simulink model "exp4simu"  (R2022b)
settings: Solver=VariableStepAuto  StartTime=0.0  StopTime=10.0  RelTol=1e-3
settings Model: Creator=16033  LastModifiedBy=16033

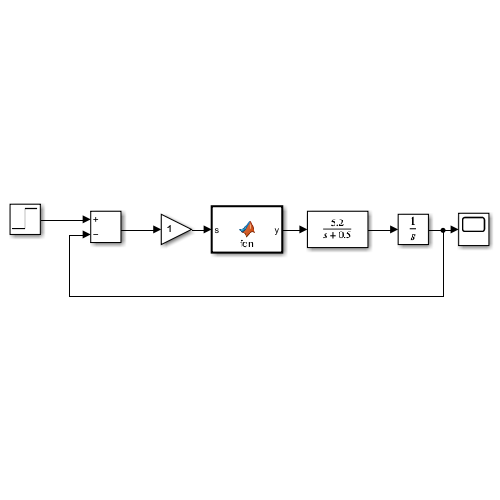
[thumbnail: Simulink's stored preview of the top-level diagram]
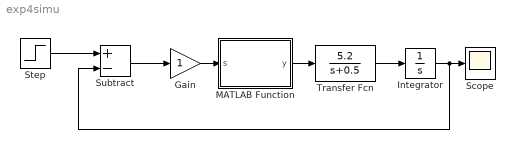
== system exp4simu ==
  Gain : Gain
  Integrator : Integrator
  MATLAB Function : MATLAB Function  TreatAsAtomicUnit=on
  Scope : Scope
  Step : Step  SampleTime=0
  Subtract : Sum  Inputs=+-
  Transfer Fcn : TransferFcn  Numerator=5.2  Denominator=[1 0.5]
  wires:
  Subtract/1 -> Gain/1
  Transfer Fcn/1 -> Integrator/1
  Integrator/1 -> Subtract/2, Scope/1
  Gain/1 -> MATLAB Function/1(s)
  MATLAB Function/1(y) -> Transfer Fcn/1
  Step/1 -> Subtract/1

== matlab function exp4simu/MATLAB Function ==
  data: s input; y output
function y = fcn(s)
    y = (s+0.02)/10*(s+0.002);
end
